simulink model "Parallel5"  (Simulink 5.0)
settings: Solver=ode45  StartTime=0.0  StopTime=10.0  RelTol=1e-3
settings Model: Creator=scaife  LastModifiedBy=scaife  ExtModeAutoUpdateStatusClock=off

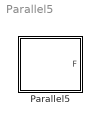
== system Parallel5 ==
  Parallel5 : Stateflow chart

== stateflow chart Parallel5 ==
  state B/ [parallel]
    on E: F;
  state A/ [parallel]
    en: E;
  events: F output EITHER_EDGE_EVENT; E local EITHER_EDGE_EVENT
